simulink model "CTC_week5"  (Simulink 9.1)
settings: Solver=ode45  StartTime=0.0  StopTime=0.4  RelTol=1e-3  EnableMultiTasking=on
values from neighbouring files (symbols this model uses):
  g = 9.81    [project_week_5.m]
  h0 = thetaA_0(1)    [project_week_5.m]
  hm = thetaA_0(1)*0.5    [project_week_5.m]
  I_lower_xx = I_C(4)    [calculate_lagrange.m]    (also in calculate_lagrange_dependent.m; calculate_lagrange_fast.m; project_week_5.m = (1/12)*m_l*L(2)^2)
  I_lower_yy = I_C(5)    [calculate_lagrange.m]    (also in calculate_lagrange_dependent.m; calculate_lagrange_fast.m; project_week_5.m = (1/12)*m_l*L(2)^2)
  I_lower_zz = I_C(6)    [calculate_lagrange.m]    (also in calculate_lagrange_dependent.m; calculate_lagrange_fast.m; project_week_5.m = I_lower_xx/10)
  I_upper_xx = I_C(1)    [calculate_lagrange.m]    (also in calculate_lagrange_dependent.m; calculate_lagrange_fast.m; project_week_5.m = (1/12)*m_u*L(1)^2)
  I_upper_yy = I_C(2)    [calculate_lagrange.m]    (also in calculate_lagrange_dependent.m; calculate_lagrange_fast.m; project_week_5.m = (1/12)*m_u*L(1)^2)
  I_upper_zz = I_C(3)    [calculate_lagrange.m]    (also in calculate_lagrange_dependent.m; calculate_lagrange_fast.m; project_week_5.m = I_upper_xx/10)
  kc = M*wc^2*sqrt(alpha)    [project_week_5.m]
  L = [0.5,1,0.3,0.8]    [plot_inverse.m]    (also in project_week_5.m; project_week_5_boundaries.m = [0.8,1,0.4,0.5]; project_week_5_symbolic.m = [L_u L_l L_e L_b])
  m_l = 0.35    [project_week_5.m]
  m_p = 1    [project_week_5.m]
  m_u = 0.35    [project_week_5.m]
  q0d = q0(ind_d)    [project_week_5.m]
  q0i = q0(ind_i)    [project_week_5.m]
  R_L1_0 = R_L1_t(:,:,1)    [calculate_acceleration.m]    (also in calculate_position.m = R_L0(:,:,1); calculate_position_dep.m = R_L0(:,:,1); calculate_position_fast.m = R_L0(:,:,1); plot_inverse.m = R_A1*rot3D_Rodrigues([0;1;0],thetaL1_y_0))
  R_L2_0 = R_L2_t(:,:,1)    [calculate_acceleration.m]    (also in calculate_position.m = R_L0(:,:,2); calculate_position_dep.m = R_L0(:,:,2); calculate_position_fast.m = R_L0(:,:,2); plot_inverse.m = R_A2*rot3D_Rodrigues([0;1;0],thetaL2_y_0))
  R_L3_0 = R_L3_t(:,:,1)    [calculate_acceleration.m]    (also in calculate_position.m = R_L0(:,:,3); calculate_position_dep.m = R_L0(:,:,3); calculate_position_fast.m = R_L0(:,:,3); plot_inverse.m = R_A3*rot3D_Rodrigues([0;1;0],thetaL3_y_0))
  ti = beta*tz    [project_week_5.m]
  tm = cycleTime    (= 0.35)    [project_week_5.m]
  tp = alpha*tz    [project_week_5.m]
  tz = 1/(wc*sqrt(alpha))    [project_week_5.m]
undefined symbols (not defined in the file or in its folder): D, thetaU_0
(part 1 of 2)
settings Model: Creator=wouterh  LastModifiedBy=rober
settings DataIOCC: LimitDataPoints=on  SignalLoggingSaveFormat=ModelDataLogs
settings OptimizationCC: ExpressionDepthLimit=2147483647  InitFltsAndDblsToZero=on
settings DebuggingCC: SolverPrmCheckMsg=warning  FcnCallInpInsideContextMsg=warning  StateNameClashWarn=warning

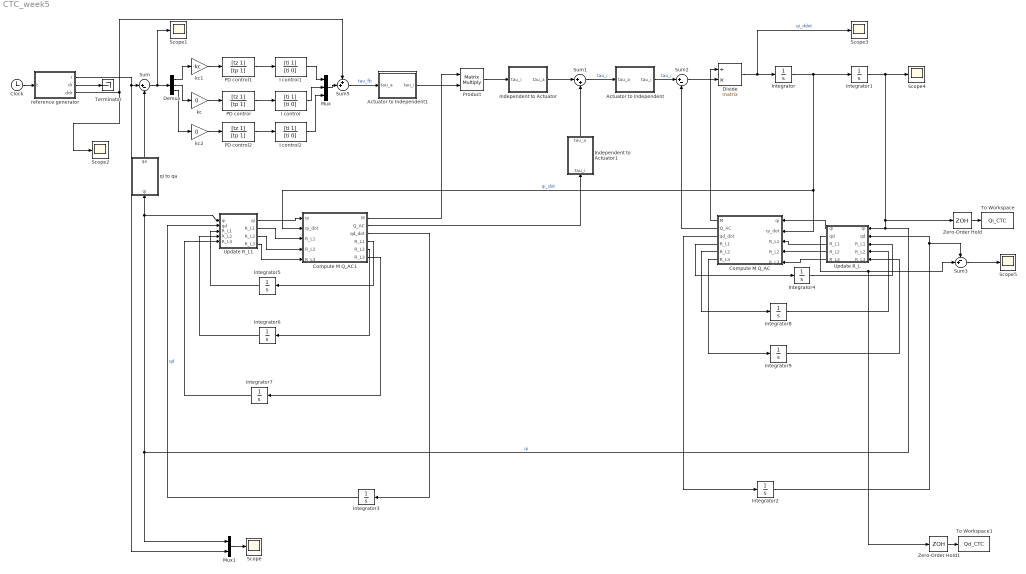
== system CTC_week5 ==
  Actuator to Independent : MATLAB Function  TreatAsAtomicUnit=on
  Actuator to Independent1 : MATLAB Function  TreatAsAtomicUnit=on
  Clock : Clock
  Compute M Q_AC : MATLAB Function  TreatAsAtomicUnit=on
  Compute M Q_AC1 : MATLAB Function  TreatAsAtomicUnit=on
  Demux : Demux  Outputs=3
  Divide : Product  Inputs=/*  Multiplication=Matrix(*)
  I control : TransferFcn  Numerator=[ti 1]  Denominator=[ti 0]
  I control1 : TransferFcn  Numerator=[ti 1]  Denominator=[ti 0]
  I control2 : TransferFcn  Numerator=[ti 1]  Denominator=[ti 0]
  Independent to Actuator : MATLAB Function  TreatAsAtomicUnit=on
  Independent to Actuator1 : MATLAB Function  TreatAsAtomicUnit=on
  Integrator : Integrator  InitialCondition=q0i
  Integrator1 : Integrator  InitialCondition=q0i
  Integrator2 : Integrator  InitialCondition=q0d
  Integrator3 : Integrator  InitialCondition=q0d
  Integrator4 : Integrator  InitialCondition=R_L1_0
  Integrator5 : Integrator  InitialCondition=R_L1_0
  Integrator6 : Integrator  InitialCondition=R_L2_0
  Integrator7 : Integrator  InitialCondition=R_L3_0
  Integrator8 : Integrator  InitialCondition=R_L2_0
  Integrator9 : Integrator  InitialCondition=R_L3_0
  Mux : Mux  Inputs=3
  Mux1 : Mux  Inputs=2
  PD control : TransferFcn  Numerator=[tz 1]  Denominator=[tp 1]
  PD control1 : TransferFcn  Numerator=[tz 1]  Denominator=[tp 1]
  PD control2 : TransferFcn  Numerator=[tz 1]  Denominator=[tp 1]
  Product : Product  Multiplication=Matrix(*)  RndMeth=Zero
  Scope{,1..5} (6 alike) : Scope
  Sum : Sum  Inputs=|+-
  Sum1 : Sum  Inputs=|++
  Sum2 : Sum  Inputs=|+-
  Sum3 : Sum  Inputs=-+|
  Sum5 : Sum  Inputs=++|
  Terminator : Terminator
  To Workspace : ToWorkspace  VariableName=Qi_CTC  SaveFormat=Timeseries  SampleTime=-1
  To Workspace1 : ToWorkspace  VariableName=Qd_CTC  SaveFormat=Timeseries  SampleTime=-1
  Update R_L : MATLAB Function  TreatAsAtomicUnit=on
  Update R_L1 : MATLAB Function  TreatAsAtomicUnit=on
  Zero-Order Hold : ZeroOrderHold  SampleTime=0.02
  Zero-Order Hold1 : ZeroOrderHold  SampleTime=0.02
  kc : Gain  Gain=0
  kc1 : Gain  Gain=-kc
  kc2 : Gain  Gain=0
  qi to qa : MATLAB Function  TreatAsAtomicUnit=on
  reference generator : MATLAB Function  TreatAsAtomicUnit=on
  wires:
  Clock/1 -> reference generator/1(t)
  reference generator/2(dr) -> Terminator/1
  reference generator/3(ddr) -> Sum5/1, Scope2/1
  Sum/1 -> Demux/1, Scope1/1
  PD control/1 -> I control/1
  Divide/1 -> Scope3/1, Integrator/1  "qi_ddot"
  Integrator/1 -> Integrator1/1, Compute M Q_AC1/2(qi_dot), Compute M Q_AC/2(qi_dot)  "qi_dot"
  Integrator1/1 -> Zero-Order Hold/1, Update R_L/1("qi "), qi to qa/1(qi), Update R_L1/1("qi "), Mux1/1, Scope4/1  "qi"
  Compute M Q_AC/1(M) -> Divide/1
  Compute M Q_AC1/2(Q_AC) -> Independent to Actuator1/1(tau_i)
  PD control1/1 -> I control1/1
  I control/1 -> Mux/2
  I control1/1 -> Mux/1
  Product/1 -> Independent to Actuator/1(tau_i)
  Mux/1 -> Sum5/2
  Sum5/1 -> Actuator to Independent1/1(tau_a)  "tau_fb"
  Mux1/1 -> Scope/1
  Compute M Q_AC/2(Q_AC) -> Sum2/2
  Compute M Q_AC/3(qd_dot) -> Integrator2/1
  Update R_L/1(qi) -> Compute M Q_AC/1(qi)
  Integrator2/1 -> Update R_L/2("qd "), Sum3/1
  kc1/1 -> PD control1/1
  Demux/1 -> kc1/1
  Demux/2 -> kc/1
  kc/1 -> PD control/1
  Sum3/1 -> Scope5/1
  reference generator/1(r) -> Mux1/2, Sum/1
  Zero-Order Hold/1 -> To Workspace/1
  Zero-Order Hold1/1 -> To Workspace1/1
  Update R_L/3(R_L1) -> Compute M Q_AC/3("R_L1 ")
  Compute M Q_AC/4(R_L1) -> Integrator4/1
  I control2/1 -> Mux/3
  kc2/1 -> PD control2/1
  PD control2/1 -> I control2/1
  Demux/3 -> kc2/1
  Update R_L1/1(qi) -> Compute M Q_AC1/1(qi)
  Update R_L1/2(R_L1) -> Compute M Q_AC1/3("R_L1 ")
  Compute M Q_AC1/4(R_L1) -> Integrator5/1
  Integrator3/1 -> Update R_L1/2(qd)  "qd"
  Sum2/1 -> Divide/2
  Actuator to Independent/1(tau_i) -> Sum2/1  "tau_i"
  qi to qa/1(qa) -> Sum/2
  Compute M Q_AC1/1(M) -> Product/1
  Sum1/1 -> Actuator to Independent/1(tau_a)  "tau_i"
  Independent to Actuator1/1(tau_a) -> Sum1/2
  Independent to Actuator/1(tau_a) -> Sum1/1
  Actuator to Independent1/1(tau_i) -> Product/2
  Compute M Q_AC1/5(R_L2) -> Integrator6/1
  Compute M Q_AC1/6(R_L3) -> Integrator7/1
  Compute M Q_AC/5(R_L2) -> Integrator8/1
  Compute M Q_AC/6(R_L3) -> Integrator9/1
  Integrator5/1 -> Update R_L1/3("R_L1 ")
  Integrator6/1 -> Update R_L1/4("R_L2 ")
  Integrator7/1 -> Update R_L1/5("R_L3 ")
  Integrator4/1 -> Update R_L/3("R_L1 ")
  Integrator8/1 -> Update R_L/4("R_L2 ")
  Integrator9/1 -> Update R_L/5("R_L3 ")
  Update R_L/2(qd) -> Zero-Order Hold1/1, Sum3/2
  Update R_L/4(R_L2) -> Compute M Q_AC/4("R_L2 ")
  Update R_L/5(R_L3) -> Compute M Q_AC/5("R_L3 ")
  Update R_L1/3(R_L2) -> Compute M Q_AC1/4("R_L2 ")
  Update R_L1/4(R_L3) -> Compute M Q_AC1/5("R_L3 ")
  Compute M Q_AC1/3(qd_dot) -> Integrator3/1

== matlab function Compute M Q_AC ==
  data: qi input double; qi_dot input double; R_L1 input double; R_L2 input double; R_L3 input double; M output double; Q_AC output double; m_u parameter double; m_p parameter double; m_l parameter double; L parameter double; D parameter double; g parameter double; qd_dot output double; R_L1 output double; I_upper_xx parameter double; I_upper_yy parameter double; I_upper_zz parameter double; I_lower_xx parameter double; I_lower_yy parameter double; I_lower_zz parameter double; thetaU_0 parameter double; R_L2 output double; R_L3 output double
function [M,Q_AC,qd_dot,R_L1,R_L2,R_L3] = fcn(qi,qi_dot,R_L1,R_L2,R_L3, m_u, m_p, m_l, L, D, g,I_upper_xx, I_upper_yy, I_upper_zz, I_lower_xx, I_lower_yy, I_lower_zz, thetaU_0)
% Compute dynamics for the system 
% Assume the model is perfect, so this is a copy past of M_Q_AC_model
% Requires running Project_week_4 first to get Mhat and Qhat


%Pre-initialise for Simulink
M=zeros(9,9);
Q_AC=zeros(9,1);
qd_dot=zeros(33,1);

%% Parameters
L_u=L(1);
L_l=L(2);
L_e=L(3);
thetaU1 = qi(1)/(+3^(1/2)/2) + thetaU_0(1); %qi()=thetaU1_x
thetaU2 = qi(4)/(-3^(1/2)/2) + thetaU_0(2); %qi()=thetaU2_x
thetaU3 = qi(8);                            %qi()=thetaU3_y
          
R_U1=rot3D_TaitByran(0, thetaU1, -2*pi/3);
R_U2=rot3D_TaitByran(0, thetaU2,  2*pi/3);
R_U3=rot3D_TaitByran(0, thetaU3,  0);
rL1_1_1 = R_L1(1,1); rL1_1_2 = R_L1(1,2); rL1_1_3 = R_L1(1,3);
rL1_2_1 = R_L1(2,1); rL1_2_2 = R_L1(2,2); rL1_2_3 = R_L1(2,3);
rL1_3_1 = R_L1(3,1); rL1_3_2 = R_L1(3,2); rL1_3_3 = R_L1(3,3);


rL2_1_1 = R_L2(1,1); rL2_1_2 = R_L2(1,2); rL2_1_3 = R_L2(1,3);
rL2_2_1 = R_L2(2,1); rL2_2_2 = R_L2(2,2); rL2_2_3 = R_L2(2,3);
rL2_3_1 = R_L2(3,1); rL2_3_2 = R_L2(3,2); rL2_3_3 = R_L2(3,3);

rL3_1_1 = R_L3(1,1); rL3_1_2 = R_L3(1,2); rL3_1_3 = R_L3(1,3);
rL3_2_1 = R_L3(2,1); rL3_2_2 = R_L3(2,2); rL3_2_3 = R_L3(2,3);
rL3_3_1 = R_L3(3,1); rL3_3_2 = R_L3(3,2); rL3_3_3 = R_L3(3,3);

%% Calculate moment inertias in the inertia frame
I_U1=R_U1*diag([I_upper_xx,I_upper_yy I_upper_zz])*R_U1.';
I_U2=R_U2*diag([I_upper_xx,I_upper_yy I_upper_zz])*R_U2.';
I_U3=R_U3*diag([I_upper_xx,I_upper_yy I_upper_zz])*R_U3.';

I_L1=R_L1*diag([I_lower_xx,I_lower_yy I_lower_zz])*R_L1.';
I_L2=R_L2*diag([I_lower_xx,I_lower_yy I_lower_zz])*R_L2.';
I_L3=R_L3*diag([I_lower_xx,I_lower_yy I_lower_zz])*R_L3.';

%% Partition into M*Qddot=[Mdd Mdi; Mid Mii]*[Qi_ddot Qd_ddot]
Mii = [I_U1 zeros(3,6);
      zeros(3,3) I_U2  zeros(3,3);
      zeros(3,6) I_U3];
Mdd = diag([0 0 0 ...
           m_u*[1 1 1]              ...
           m_l*[1 1 1] I_lower_xx I_lower_yy I_lower_zz ...
           m_u*[1 1 1]              ...
           m_l*[1 1 1] I_lower_xx I_lower_yy I_lower_zz ...
           m_u*[1 1 1]              ...
           m_l*[1 1 1] I_lower_xx I_lower_yy I_lower_zz ...
           m_p*[1 1 1] ]); 
% Correct Mdd
Mdd(10:12,10:12)=I_L1;
Mdd(19:21,19:21)=I_L2;
Mdd(28:30,28:30)=I_L3;
  
Mdi = zeros(33,9);
Mid = zeros(9,33);

%% function Jacobian_d = Jacobian_dNumeric(L_l,rL1_1_1,rL1_1_2,rL1_2_1,rL1_2_2,rL1_3_1,rL1_3_2,rL2_1_1,rL2_1_2,rL2_2_1,rL2_2_2,rL2_3_1,rL2_3_2,rL3_1_1,rL3_1_2,rL3_2_1,rL3_2_2,rL3_3_1,rL3_3_2)
%    This function was generated by the Symbolic Math Toolbox version 8.0.
t2 = L_l.*rL1_1_2.*rL1_2_1.*(1.0./2.0);
t3 = L_l.*rL1_1_2.*rL1_3_1.*(1.0./2.0);
t4 = L_l.*rL1_2_2.*rL1_3_1.*(1.0./2.0);
t5 = L_l.*rL1_1_1.*rL1_2_2.*(1.0./2.0);
t6 = L_l.*rL1_1_1.*rL1_3_2.*(1.0./2.0);
t7 = -t2+t5;
t8 = L_l.*rL1_2_1.*rL1_3_2.*(1.0./2.0);
t9 = -t3+t6;
t10 = -t4+t8;
t11 = L_l.*rL2_1_2.*rL2_2_1.*(1.0./2.0);
t12 = L_l.*rL2_1_2.*rL2_3_1.*(1.0./2.0);
t13 = L_l.*rL2_2_2.*rL2_3_1.*(1.0./2.0);
t14 = L_l.*rL2_1_1.*rL2_2_2.*(1.0./2.0);
t15 = L_l.*rL2_1_1.*rL2_3_2.*(1.0./2.0);
t16 = -t11+t14;
t17 = L_l.*rL2_2_1.*rL2_3_2.*(1.0./2.0);
t18 = -t12+t15;
t19 = -t13+t17;
t20 = L_l.*rL3_1_2.*rL3_2_1.*(1.0./2.0);
t21 = L_l.*rL3_1_2.*rL3_3_1.*(1.0./2.0);
t22 = L_l.*rL3_2_2.*rL3_3_1.*(1.0./2.0);
t23 = L_l.*rL3_1_1.*rL3_2_2.*(1.0./2.0);
t24 = L_l.*rL3_1_1.*rL3_3_2.*(1.0./2.0);
t25 = -t20+t23;
t26 = L_l.*rL3_2_1.*rL3_3_2.*(1.0./2.0);
t27 = -t21+t24;
t28 = -t22+t26;
t29 = sqrt(2.0);
t30 = sqrt(3.0);
Jacobian_d = reshape([1.0,0.0,0.0,0.0,0.0,0.0,0.0,0.0,0.0,1.0,0.0,0.0,0.0,0.0,0.0,0.0,0.0,0.0,1.0,0.0,0.0,0.0,0.0,0.0,0.0,0.0,0.0,1.0,0.0,0.0,0.0,0.0,0.0,0.0,1.0,0.0,0.0,0.0,0.0,0.0,0.0,0.0,0.0,1.0,0.0,0.0,0.0,0.0,0.0,0.0,0.0,0.0,1.0,0.0,0.0,0.0,0.0,0.0,0.0,0.0,0.0,1.0,0.0,0.0,0.0,0.0,0.0,0.0,1.0,0.0,0.0,0.0,0.0,0.0,0.0,0.0,0.0,1.0,0.0,0.0,0.0,0.0,0.0,0.0,0.0,0.0,1.0,0.0,0.0,0.0,0.0,0.0,0.0,0.0,0.0,1.0,0.0,0.0,0.0,-1.0,0.0,0.0,1.0,0.0,0.0,0.0,0.0,0.0,0.0,0.0,0.0,0.0,0.0,0.0,0.0,0.0,0.0,0.0,0.0,0.0,0.0,0.0,0.0,0.0,0.0,0.0,0.0,0.0,0.0,0.0,0.0,0.0,0.0,-1.0,0.0,0.0,1.0,0.0,0.0,0.0,0.0,0.0,0.0,0.0,0.0,0.0,0.0,0.0,0.0,0.0,0.0,0.0,0.0,0.0,0.0,0.0,0.0,0.0,0.0,0.0,0.0,0.0,0.0,0.0,0.0,0.0,0.0,-1.0,0.0,0.0,1.0,0.0,0.0,0.0,0.0,0.0,0.0,0.0,0.0,0.0,0.0,0.0,0.0,0.0,0.0,0.0,0.0,0.0,0.0,0.0,0.0,0.0,0.0,0.0,0.0,0.0,0.0,0.0,0.0,0.0,0.0,-1.0,0.0,0.0,1.0,0.0,0.0,0.0,0.0,0.0,0.0,0.0,0.0,0.0,0.0,0.0,0.0,0.0,0.0,0.0,0.0,0.0,0.0,0.0,0.0,0.0,0.0,0.0,0.0,0.0,0.0,0.0,0.0,0.0,0.0,-1.0,0.0,0.0,1.0,0.0,0.0,0.0,0.0,0.0,0.0,0.0,0.0,0.0,0.0,0.0,0.0,0.0,0.0,0.0,0.0,0.0,0.0,0.0,0.0,0.0,0.0,0.0,0.0,0.0,0.0,0.0,0.0,0.0,0.0,-1.0,0.0,0.0,1.0,0.0,0.0,0.0,0.0,0.0,0.0,0.0,0.0,0.0,0.0,0.0,0.0,0.0,0.0,0.0,0.0,0.0,0.0,0.0,0.0,0.0,0.0,0.0,0.0,0.0,0.0,0.0,0.0,t7,t9,0.0,t7,t9,0.0,0.0,0.0,0.0,0.0,0.0,0.0,0.0,0.0,0.0,0.0,0.0,0.0,0.0,0.0,0.0,0.0,0.0,0.0,0.0,0.0,rL1_2_2.*t29.*(-1.0./2.0)+rL1_3_2.*t29.*t30.*(1.0./4.0),0.0,0.0,0.0,0.0,0.0,t2-L_l.*rL1_1_1.*rL1_2_2.*(1.0./2.0),0.0,t10,t2-t5,0.0,t10,0.0,0.0,0.0,0.0,0.0,0.0,0.0,0.0,0.0,0.0,0.0,0.0,0.0,0.0,0.0,0.0,0.0,0.0,0.0,0.0,0.0,rL1_1_2.*t29.*(1.0./2.0)-rL1_3_2.*t29.*(1.0./4.0),0.0,0.0,0.0,0.0,0.0,t3-L_l.*rL1_1_1.*rL1_3_2.*(1.0./2.0),t4-L_l.*rL1_2_1.*rL1_3_2.*(1.0./2.0),0.0,t3-t6,t4-t8,0.0,0.0,0.0,0.0,0.0,0.0,0.0,0.0,0.0,0.0,0.0,0.0,0.0,0.0,0.0,0.0,0.0,0.0,0.0,0.0,0.0,0.0,rL1_2_2.*t29.*(1.0./4.0)-rL1_1_2.*t29.*t30.*(1.0./4.0),0.0,0.0,0.0,0.0,0.0,0.0,0.0,0.0,0.0,0.0,0.0,-1.0,0.0,0.0,1.0,0.0,0.0,0.0,0.0,0.0,0.0,0.0,0.0,0.0,0.0,0.0,0.0,0.0,0.0,0.0,0.0,0.0,0.0,0.0,0.0,0.0,0.0,0.0,0.0,0.0,0.0,0.0,0.0,0.0,0.0,-1.0,0.0,0.0,1.0,0.0,0.0,0.0,0.0,0.0,0.0,0.0,0.0,0.0,0.0,0.0,0.0,0.0,0.0,0.0,0.0,0.0,0.0,0.0,0.0,0.0,0.0,0.0,0.0,0.0,0.0,0.0,0.0,0.0,0.0,-1.0,0.0,0.0,1.0,0.0,0.0,0.0,0.0,0.0,0.0,0.0,0.0,0.0,0.0,0.0,0.0,0.0,0.0,0.0,0.0,0.0,0.0,0.0,0.0,0.0,0.0,0.0,0.0,0.0,0.0,0.0,0.0,0.0,0.0,-1.0,0.0,0.0,1.0,0.0,0.0,0.0,0.0,0.0,0.0,0.0,0.0,0.0,0.0,0.0,0.0,0.0,0.0,0.0,0.0,0.0,0.0,0.0,0.0,0.0,0.0,0.0,0.0,0.0,0.0,0.0,0.0,0.0,0.0,-1.0,0.0,0.0,1.0,0.0,0.0,0.0,0.0,0.0,0.0,0.0,0.0,0.0,0.0,0.0,0.0,0.0,0.0,0.0,0.0,0.0,0.0,0.0,0.0,0.0,0.0,0.0,0.0,0.0,0.0,0.0,0.0,0.0,0.0,-1.0,0.0,0.0,1.0,0.0,0.0,0.0,0.0,0.0,0.0,0.0,0.0,0.0,0.0,0.0,0.0,0.0,0.0,0.0,0.0,0.0,0.0,0.0,0.0,0.0,0.0,0.0,0.0,0.0,0.0,0.0,0.0,t16,t18,0.0,t16,t18,0.0,0.0,0.0,0.0,0.0,0.0,0.0,0.0,0.0,0.0,0.0,0.0,0.0,rL2_2_2.*t29.*(-1.0./2.0)-rL2_3_2.*t29.*t30.*(1.0./4.0),0.0,0.0,0.0,0.0,0.0,0.0,0.0,0.0,0.0,0.0,0.0,0.0,0.0,t11-L_l.*rL2_1_1.*rL2_2_2.*(1.0./2.0),0.0,t19,t11-t14,0.0,t19,0.0,0.0,0.0,0.0,0.0,0.0,0.0,0.0,0.0,0.0,0.0,0.0,0.0,rL2_1_2.*t29.*(1.0./2.0)-rL2_3_2.*t29.*(1.0./4.0),0.0,0.0,0.0,0.0,0.0,0.0,0.0,0.0,0.0,0.0,0.0,0.0,0.0,t12-L_l.*rL2_1_1.*rL2_3_2.*(1.0./2.0),t13-L_l.*rL2_2_1.*rL2_3_2.*(1.0./2.0),0.0,t12-t15,t13-t17,0.0,0.0,0.0,0.0,0.0,0.0,0.0,0.0,0.0,0.0,0.0,0.0,0.0,0.0,rL2_2_2.*t29.*(1.0./4.0)+rL2_1_2.*t29.*t30.*(1.0./4.0),0.0,0.0,0.0,0.0,0.0,0.0,0.0,0.0,0.0,0.0,0.0,0.0,0.0,0.0,0.0,0.0,0.0,0.0,0.0,-1.0,0.0,0.0,1.0,0.0,0.0,0.0,0.0,0.0,0.0,0.0,0.0,0.0,0.0,0.0,0.0,0.0,0.0,0.0,0.0,0.0,0.0,0.0,0.0,0.0,0.0,0.0,0.0,0.0,0.0,0.0,0.0,0.0,0.0,-1.0,0.0,0.0,1.0,0.0,0.0,0.0,0.0,0.0,0.0,0.0,0.0,0.0,0.0,0.0,0.0,0.0,0.0,0.0,0.0,0.0,0.0,0.0,0.0,0.0,0.0,0.0,0.0,0.0,0.0,0.0,0.0,0.0,0.0,-1.0,0.0,0.0,1.0,0.0,0.0,0.0,0.0,0.0,0.0,0.0,0.0,0.0,0.0,0.0,0.0,0.0,0.0,0.0,0.0,0.0,0.0,0.0,0.0,0.0,0.0,0.0,0.0,0.0,0.0,0.0,0.0,0.0,0.0,-1.0,0.0,0.0,1.0,0.0,0.0,0.0,0.0,0.0,0.0,0.0,0.0,0.0,0.0,0.0,0.0,0.0,0.0,0.0,0.0,0.0,0.0,0.0,0.0,0.0,0.0,0.0,0.0,0.0,0.0,0.0,0.0,0.0,0.0,-1.0,0.0,0.0,1.0,0.0,0.0,0.0,0.0,0.0,0.0,0.0,0.0,0.0,0.0,0.0,0.0,0.0,0.0,0.0,0.0,0.0,0.0,0.0,0.0,0.0,0.0,0.0,0.0,0.0,0.0,0.0,0.0,0.0,0.0,-1.0,0.0,0.0,1.0,0.0,0.0,0.0,0.0,0.0,0.0,0.0,0.0,0.0,0.0,0.0,0.0,0.0,0.0,0.0,0.0,0.0,0.0,0.0,0.0,0.0,0.0,0.0,0.0,0.0,0.0,0.0,0.0,t25,t27,0.0,t25,t27,0.0,0.0,0.0,0.0,0.0,rL3_2_2.*t29.*(-1.0./2.0),0.0,0.0,0.0,0.0,0.0,0.0,0.0,0.0,0.0,0.0,0.0,0.0,0.0,0.0,0.0,0.0,0.0,0.0,0.0,0.0,0.0,t20-L_l.*rL3_1_1.*rL3_2_2.*(1.0./2.0),0.0,t28,t20-t23,0.0,t28,0.0,0.0,0.0,0.0,0.0,rL3_1_2.*t29.*(1.0./2.0)+rL3_3_2.*t29.*(1.0./2.0),0.0,0.0,0.0,0.0,0.0,0.0,0.0,0.0,0.0,0.0,0.0,0.0,0.0,0.0,0.0,0.0,0.0,0.0,0.0,0.0,0.0,t21-L_l.*rL3_1_1.*rL3_3_2.*(1.0./2.0),t22-L_l.*rL3_2_1.*rL3_3_2.*(1.0./2.0),0.0,t21-t24,t22-t26,0.0,0.0,0.0,0.0,0.0,0.0,rL3_2_2.*t29.*(-1.0./2.0),0.0,0.0,0.0,0.0,0.0,0.0,-1.0,0.0,0.0,0.0,0.0,0.0,0.0,0.0,0.0,-1.0,0.0,0.0,0.0,0.0,0.0,0.0,0.0,0.0,-1.0,0.0,0.0,0.0,0.0,0.0,0.0,0.0,0.0,0.0,0.0,0.0,0.0,0.0,0.0,0.0,-1.0,0.0,0.0,0.0,0.0,0.0,0.0,0.0,0.0,-1.0,0.0,0.0,0.0,0.0,0.0,0.0,0.0,0.0,-1.0,0.0,0.0,0.0,0.0,0.0,0.0,0.0,0.0,0.0,0.0,0.0,0.0,0.0,0.0,0.0,-1.0,0.0,0.0,0.0,0.0,0.0,0.0,0.0,0.0,-1.0,0.0,0.0,0.0,0.0,0.0,0.0,0.0,0.0,-1.0,0.0,0.0,0.0,0.0,0.0,0.0],[33,33]);

%% function Jacobian_i = Jacobian_iNumeric(L_u,thetaU1,thetaU2,thetaU3)
t2 = cos(thetaU1);
t3 = sin(thetaU1);
t4 = sqrt(3.0);
t5 = L_u.*t3.*(1.0./4.0);
t6 = L_u.*t2.*(1.0./2.0);
t7 = L_u.*t3.*t4.*(1.0./4.0);
t8 = cos(thetaU2);
t9 = sin(thetaU2);
t10 = L_u.*t4.*t9.*(1.0./4.0);
t11 = L_u.*t9.*(1.0./4.0);
t12 = L_u.*t8.*(1.0./2.0);
t13 = cos(thetaU3);
t14 = sin(thetaU3);
t15 = L_u.*t13.*(1.0./2.0);
t16 = L_u.*t14.*(1.0./2.0);
Jacobian_i = reshape([0.0,t6,t7,0.0,t6,t7,0.0,0.0,0.0,0.0,0.0,0.0,0.0,0.0,0.0,0.0,0.0,0.0,0.0,0.0,0.0,0.0,0.0,0.0,0.0,0.0,0.0,0.0,0.0,0.0,0.0,0.0,0.0,L_u.*t2.*(-1.0./2.0),0.0,-t5,-t6,0.0,-t5,0.0,0.0,0.0,0.0,0.0,0.0,0.0,0.0,0.0,0.0,0.0,0.0,0.0,0.0,0.0,0.0,0.0,0.0,0.0,0.0,0.0,0.0,0.0,0.0,0.0,0.0,0.0,L_u.*t3.*t4.*(-1.0./4.0),t5,0.0,-t7,t5,0.0,0.0,0.0,0.0,0.0,0.0,0.0,0.0,0.0,0.0,0.0,0.0,0.0,0.0,0.0,0.0,0.0,0.0,0.0,0.0,0.0,0.0,0.0,0.0,0.0,0.0,0.0,0.0,0.0,0.0,0.0,0.0,0.0,0.0,0.0,0.0,0.0,0.0,t12,-t10,0.0,t12,-t10,0.0,0.0,0.0,0.0,0.0,0.0,0.0,0.0,0.0,0.0,0.0,0.0,0.0,0.0,0.0,0.0,0.0,0.0,0.0,0.0,0.0,0.0,0.0,0.0,0.0,0.0,0.0,L_u.*t8.*(-1.0./2.0),0.0,-t11,-t12,0.0,-t11,0.0,0.0,0.0,0.0,0.0,0.0,0.0,0.0,0.0,0.0,0.0,0.0,0.0,0.0,0.0,0.0,0.0,0.0,0.0,0.0,0.0,0.0,0.0,0.0,0.0,0.0,0.0,t10,t11,0.0,t10,t11,0.0,0.0,0.0,0.0,0.0,0.0,0.0,0.0,0.0,0.0,0.0,0.0,0.0,0.0,0.0,0.0,0.0,0.0,0.0,0.0,0.0,0.0,0.0,0.0,0.0,0.0,0.0,0.0,0.0,0.0,0.0,0.0,0.0,0.0,0.0,0.0,0.0,0.0,t15,0.0,0.0,t15,0.0,0.0,0.0,0.0,0.0,0.0,0.0,0.0,0.0,0.0,0.0,0.0,0.0,0.0,0.0,0.0,0.0,0.0,0.0,0.0,0.0,0.0,0.0,0.0,0.0,0.0,0.0,0.0,L_u.*t13.*(-1.0./2.0),0.0,t16,-t15,0.0,t16,0.0,0.0,0.0,0.0,0.0,0.0,0.0,0.0,0.0,0.0,0.0,0.0,0.0,0.0,0.0,0.0,0.0,0.0,0.0,0.0,0.0,0.0,0.0,0.0,0.0,0.0,0.0,0.0,L_u.*t14.*(-1.0./2.0),0.0,0.0,-t16,0.0,0.0,0.0,0.0,0.0,0.0,0.0,0.0,0.0,0.0],[33,9]);

%% Compute dependent velocities
P = Jacobian_d\Jacobian_i;
Phi_t=zeros(33,1);
qd_dot = -P*qi_dot-Jacobian_d\Phi_t;

qdot=[qd_dot(1:6); qi_dot(1:3);qd_dot(7:16);qi_dot(4:6);qd_dot(17:26);qi_dot(7:9);qd_dot(27:33)];
qdot1=qdot(1);
qdot2=qdot(2);
qdot3=qdot(3);
qdot4=qdot(4);
qdot5=qdot(5);
qdot6=qdot(6);
qdot7=qdot(7);
qdot8=qdot(8);
qdot9=qdot(9);
qdot10=qdot(10);
qdot11=qdot(11);
qdot12=qdot(12);
qdot13=qdot(13);
qdot14=qdot(14);
qdot15=qdot(15);
qdot16=qdot(16);
qdot17=qdot(17);
qdot18=qdot(18);
qdot19=qdot(19);
qdot20=qdot(20);
qdot21=qdot(21);
qdot22=qdot(22);
qdot23=qdot(23);
qdot24=qdot(24);
qdot25=qdot(25);
qdot26=qdot(26);
qdot27=qdot(27);
qdot28=qdot(28);
qdot29=qdot(29);
qdot30=qdot(30);
qdot31=qdot(31);
qdot32=qdot(32);
qdot33=qdot(33);
qdot34=qdot(34);
qdot35=qdot(35);
qdot36=qdot(36);
qdot37=qdot(37);
qdot38=qdot(38);
qdot39=qdot(39);
qdot40=qdot(40);
qdot41=qdot(41);
qdot42=qdot(42);
%% function Gamma_without_driving = Gamma_without_drivingNumeric(L_l,L_u,qdot7,qdot8,qdot9,qdot13,qdot14,qdot15,qdot19,qdot20,qdot21,qdot25,qdot26,qdot27,qdot31,qdot32,qdot33,qdot37,qdot38,qdot39,rL1_1_1,rL1_1_2,rL1_1_3,rL1_2_1,rL1_2_2,rL1_2_3,rL1_3_1,rL1_3_2,rL1_3_3,rL2_1_1,rL2_1_2,rL2_1_3,rL2_2_1,rL2_2_2,rL2_2_3,rL2_3_1,rL2_3_2,rL2_3_3,rL3_1_1,rL3_1_2,rL3_1_3,rL3_2_1,rL3_2_2,rL3_2_3,rL3_3_1,rL3_3_2,rL3_3_3,thetaU1,thetaU2,thetaU3)
%    This function was generated by the Symbolic Math Toolbox version 8.0.
t2 = sqrt(3.0);
t3 = cos(thetaU1);
t4 = sin(thetaU1);
t5 = qdot8.*t4;
t22 = qdot9.*t2.*t3.*(1.0./2.0);
t6 = t5-t22;
t7 = L_u.*qdot9.*t2.*t3.*(1.0./8.0);
t8 = qdot7.*t4;
t33 = qdot9.*t3.*(1.0./2.0);
t9 = t8-t33;
t10 = qdot9.^2;
t11 = qdot8.*t3.*(1.0./2.0);
t38 = qdot7.*t2.*t3.*(1.0./2.0);
t12 = t11-t38;
t13 = qdot7.*(1.0./2.0);
t14 = qdot8.*t2.*(1.0./2.0);
t15 = t13+t14;
t16 = qdot15.*rL1_2_1;
t20 = qdot14.*rL1_3_1;
t17 = t16-t20;
t18 = qdot15.*rL1_2_2;
t21 = qdot14.*rL1_3_2;
t19 = t18-t21;
t23 = L_u.*qdot9.*t3.*(1.0./8.0);
t24 = t23-L_u.*t2.*t6.*(1.0./4.0);
t25 = L_u.*t6.*(1.0./4.0);
t26 = t7+t25;
t27 = qdot15.*rL1_1_1;
t31 = qdot13.*rL1_3_1;
t28 = t27-t31;
t29 = qdot15.*rL1_1_2;
t32 = qdot13.*rL1_3_2;
t30 = t29-t32;
t34 = L_u.*t2.*t9.*(1.0./4.0);
t35 = t7+t34;
t36 = L_u.*t9.*(1.0./4.0);
t37 = qdot8.*(t36-L_u.*qdot9.*t3.*(3.0./8.0));
t39 = L_u.*t2.*t12.*(1.0./4.0);
t40 = t39-L_u.*t3.*t15.*(1.0./4.0);
t41 = L_u.*t12.*(1.0./4.0);
t42 = L_u.*t2.*t3.*t15.*(1.0./4.0);
t43 = t41+t42;
t44 = qdot8.*t43;
t45 = qdot14.*rL1_1_1;
t49 = qdot13.*rL1_2_1;
t46 = t45-t49;
t47 = qdot14.*rL1_1_2;
t50 = qdot13.*rL1_2_2;
t48 = t47-t50;
t51 = L_u.*qdot9.*t4.*t15.*(1.0./2.0);
t52 = L_l.*rL1_1_2.*t17.*(1.0./2.0);
t53 = t52-L_l.*rL1_1_1.*t19.*(1.0./2.0);
t54 = qdot13.*t53;
t55 = L_l.*rL1_2_2.*t17.*(1.0./2.0);
t56 = t55-L_l.*rL1_2_1.*t19.*(1.0./2.0);
t57 = qdot14.*t56;
t58 = L_l.*rL1_3_2.*t17.*(1.0./2.0);
t59 = t58-L_l.*rL1_3_1.*t19.*(1.0./2.0);
t60 = qdot15.*t59;
t61 = L_l.*rL1_1_2.*t28.*(1.0./2.0);
t62 = t61-L_l.*rL1_1_1.*t30.*(1.0./2.0);
t63 = L_l.*rL1_2_2.*t28.*(1.0./2.0);
t64 = t63-L_l.*rL1_2_1.*t30.*(1.0./2.0);
t65 = L_l.*rL1_3_2.*t28.*(1.0./2.0);
t66 = t65-L_l.*rL1_3_1.*t30.*(1.0./2.0);
t67 = L_l.*rL1_1_2.*t46.*(1.0./2.0);
t68 = t67-L_l.*rL1_1_1.*t48.*(1.0./2.0);
t69 = qdot13.*t68;
t70 = L_l.*rL1_2_2.*t46.*(1.0./2.0);
t71 = t70-L_l.*rL1_2_1.*t48.*(1.0./2.0);
t72 = qdot14.*t71;
t73 = L_l.*rL1_3_2.*t46.*(1.0./2.0);
t74 = t73-L_l.*rL1_3_1.*t48.*(1.0./2.0);
t75 = qdot15.*t74;
t76 = cos(thetaU2);
t77 = sin(thetaU2);
t78 = qdot20.*t77;
t79 = qdot21.*t2.*t76.*(1.0./2.0);
t80 = t78+t79;
t81 = qdot19.*t77;
t107 = qdot21.*t76.*(1.0./2.0);
t82 = t81-t107;
t83 = qdot21.^2;
t84 = qdot20.*t76.*(1.0./2.0);
t85 = qdot19.*t2.*t76.*(1.0./2.0);
t86 = t84+t85;
t87 = qdot19.*(1.0./2.0);
t89 = qdot20.*t2.*(1.0./2.0);
t88 = t87-t89;
t90 = qdot27.*rL2_2_1;
t94 = qdot26.*rL2_3_1;
t91 = t90-t94;
t92 = qdot27.*rL2_2_2;
t95 = qdot26.*rL2_3_2;
t93 = t92-t95;
t96 = L_u.*t2.*t80.*(1.0./4.0);
t97 = L_u.*qdot21.*t76.*(1.0./8.0);
t98 = t96+t97;
t99 = L_u.*t80.*(1.0./4.0);
t100 = L_u.*qdot21.*t2.*t76.*(1.0./8.0);
t101 = qdot27.*rL2_1_1;
t105 = qdot25.*rL2_3_1;
t102 = t101-t105;
t103 = qdot27.*rL2_1_2;
t106 = qdot25.*rL2_3_2;
t104 = t103-t106;
t108 = L_u.*t2.*t82.*(1.0./4.0);
t109 = qdot19.*(t100+t108);
t110 = L_u.*t82.*(1.0./4.0);
t111 = qdot20.*(t110-L_u.*qdot21.*t76.*(3.0./8.0));
t112 = L_u.*t2.*t77.*t83.*(1.0./4.0);
t113 = L_u.*t2.*t86.*(1.0./4.0);
t114 = L_u.*t76.*t88.*(1.0./4.0);
t115 = t113+t114;
t116 = qdot19.*t115;
t117 = L_u.*t86.*(1.0./4.0);
t118 = t117-L_u.*t2.*t76.*t88.*(1.0./4.0);
t119 = qdot20.*t118;
t120 = qdot26.*rL2_1_1;
t124 = qdot25.*rL2_2_1;
t121 = t120-t124;
t122 = qdot26.*rL2_1_2;
t125 = qdot25.*rL2_2_2;
t123 = t122-t125;
t126 = L_u.*qdot21.*t77.*t88.*(1.0./2.0);
t127 = L_l.*rL2_1_2.*t91.*(1.0./2.0);
t128 = t127-L_l.*rL2_1_1.*t93.*(1.0./2.0);
t129 = qdot25.*t128;
t130 = L_l.*rL2_2_2.*t91.*(1.0./2.0);
t131 = t130-L_l.*rL2_2_1.*t93.*(1.0./2.0);
t132 = qdot26.*t131;
t133 = L_l.*rL2_3_2.*t91.*(1.0./2.0);
t134 = t133-L_l.*rL2_3_1.*t93.*(1.0./2.0);
t135 = qdot27.*t134;
t136 = L_l.*rL2_1_2.*t102.*(1.0./2.0);
t137 = t136-L_l.*rL2_1_1.*t104.*(1.0./2.0);
t138 = L_l.*rL2_2_2.*t102.*(1.0./2.0);
t139 = t138-L_l.*rL2_2_1.*t104.*(1.0./2.0);
t140 = L_l.*rL2_3_2.*t102.*(1.0./2.0);
t141 = t140-L_l.*rL2_3_1.*t104.*(1.0./2.0);
t142 = L_l.*rL2_1_2.*t121.*(1.0./2.0);
t143 = t142-L_l.*rL2_1_1.*t123.*(1.0./2.0);
t144 = qdot25.*t143;
t145 = L_l.*rL2_2_2.*t121.*(1.0./2.0);
t146 = t145-L_l.*rL2_2_1.*t123.*(1.0./2.0);
t147 = qdot26.*t146;
t148 = L_l.*rL2_3_2.*t121.*(1.0./2.0);
t149 = t148-L_l.*rL2_3_1.*t123.*(1.0./2.0);
t150 = qdot27.*t149;
t151 = sin(thetaU3);
t152 = cos(thetaU3);
t153 = qdot32.^2;
t154 = qdot39.*rL3_2_1;
t158 = qdot38.*rL3_3_1;
t155 = t154-t158;
t156 = qdot39.*rL3_2_2;
t159 = qdot38.*rL3_3_2;
t157 = t156-t159;
t160 = L_u.*t151.*t153.*(1.0./2.0);
t161 = qdot33.^2;
t162 = L_u.*t151.*t161.*(1.0./2.0);
t163 = qdot39.*rL3_1_1;
t167 = qdot37.*rL3_3_1;
t164 = t163-t167;
t165 = qdot39.*rL3_1_2;
t168 = qdot37.*rL3_3_2;
t166 = t165-t168;
t169 = qdot33.*t152;
t170 = qdot31.*t151;
t171 = t169+t170;
t172 = qdot38.*rL3_1_1;
t176 = qdot37.*rL3_2_1;
t173 = t172-t176;
t174 = qdot38.*rL3_1_2;
t177 = qdot37.*rL3_2_2;
t175 = t174-t177;
t178 = qdot31.^2;
t179 = L_u.*t152.*t178.*(1.0./2.0);
t180 = L_u.*t152.*t153.*(1.0./2.0);
t181 = L_l.*rL3_1_2.*t155.*(1.0./2.0);
t182 = t181-L_l.*rL3_1_1.*t157.*(1.0./2.0);
t183 = qdot37.*t182;
t184 = L_l.*rL3_2_2.*t155.*(1.0./2.0);
t185 = t184-L_l.*rL3_2_1.*t157.*(1.0./2.0);
t186 = qdot38.*t185;
t187 = L_l.*rL3_3_2.*t155.*(1.0./2.0);
t188 = t187-L_l.*rL3_3_1.*t157.*(1.0./2.0);
t189 = qdot39.*t188;
t190 = L_l.*rL3_1_2.*t164.*(1.0./2.0);
t191 = t190-L_l.*rL3_1_1.*t166.*(1.0./2.0);
t192 = L_l.*rL3_2_2.*t164.*(1.0./2.0);
t193 = t192-L_l.*rL3_2_1.*t166.*(1.0./2.0);
t194 = L_l.*rL3_3_2.*t164.*(1.0./2.0);
t195 = t194-L_l.*rL3_3_1.*t166.*(1.0./2.0);
t196 = L_l.*rL3_1_2.*t173.*(1.0./2.0);
t197 = t196-L_l.*rL3_1_1.*t175.*(1.0./2.0);
t198 = qdot37.*t197;
t199 = L_l.*rL3_2_2.*t173.*(1.0./2.0);
t200 = t199-L_l.*rL3_2_1.*t175.*(1.0./2.0);
t201 = qdot38.*t200;
t202 = L_l.*rL3_3_2.*t173.*(1.0./2.0);
t203 = t202-L_l.*rL3_3_1.*t175.*(1.0./2.0);
t204 = qdot39.*t203;
t205 = sqrt(2.0);
t206 = t16-qdot13.*rL1_2_3;
t207 = qdot13.*rL1_3_3;
t208 = t207-qdot15.*rL1_3_1;
t209 = t101-qdot25.*rL2_1_3;
t210 = t90-qdot25.*rL2_2_3;
t211 = qdot25.*rL2_3_3;
t212 = t211-qdot27.*rL2_3_1;
t213 = t154-qdot37.*rL3_2_3;
Gamma_without_driving = [-qdot7.*t24-qdot8.*t26-L_u.*t4.*t10.*(1.0./4.0);t37-qdot7.*t35-L_u.*t2.*t4.*t10.*(1.0./4.0);t44+t51-qdot7.*t40;t54+t57+t60-qdot7.*t24-qdot8.*t26-L_u.*t4.*t10.*(1.0./4.0);t37-qdot7.*t35-qdot13.*t62-qdot14.*t64-qdot15.*t66-L_u.*t2.*t4.*t10.*(1.0./4.0);t44+t51+t69+t72+t75-qdot7.*t40;t54+t57+t60;-qdot13.*t62-qdot14.*t64-qdot15.*t66;t69+t72+t75;-qdot19.*t98-qdot20.*(t99-L_u.*qdot21.*t2.*t76.*(1.0./8.0))-L_u.*t77.*t83.*(1.0./4.0);t109+t111+t112;t116+t119+t126;t129+t132+t135-qdot19.*t98-qdot20.*(t99-t100)-L_u.*t77.*t83.*(1.0./4.0);t109+t111+t112-qdot25.*t137-qdot26.*t139-qdot27.*t141;t116+t119+t126+t144+t147+t150;t129+t132+t135;-qdot25.*t137-qdot26.*t139-qdot27.*t141;t144+t147+t150;t160+t162-L_u.*qdot31.*qdot33.*t152.*(1.0./2.0);L_u.*qdot32.*t171.*(-1.0./2.0);t179+t180-L_u.*qdot31.*qdot33.*t151.*(1.0./2.0);t160+t162+t183+t186+t189-L_u.*qdot31.*qdot33.*t152.*(1.0./2.0);-qdot37.*t191-qdot38.*t193-qdot39.*t195-L_u.*qdot32.*t171.*(1.0./2.0);t179+t180+t198+t201+t204-L_u.*qdot31.*qdot33.*t151.*(1.0./2.0);t183+t186+t189;-qdot37.*t191-qdot38.*t193-qdot39.*t195;t198+t201+t204;0.0;0.0;0.0;-qdot13.*(t205.*t206.*(1.0./2.0)+t2.*t205.*t208.*(1.0./4.0))+qdot14.*(t205.*t208.*(1.0./4.0)+t205.*(t27-qdot13.*rL1_1_3).*(1.0./2.0))+qdot15.*(t205.*t206.*(1.0./4.0)-t2.*t205.*(t27-qdot13.*rL1_1_3).*(1.0./4.0));-qdot25.*(t205.*t210.*(1.0./2.0)-t2.*t205.*t212.*(1.0./4.0))+qdot27.*(t205.*t210.*(1.0./4.0)+t2.*t205.*t209.*(1.0./4.0))+qdot26.*(t205.*t209.*(1.0./2.0)+t205.*t212.*(1.0./4.0));-qdot38.*(t205.*(qdot37.*rL3_3_3-qdot39.*rL3_3_1).*(1.0./2.0)-t205.*(t163-qdot37.*rL3_1_3).*(1.0./2.0))-qdot37.*t205.*t213.*(1.0./2.0)-qdot39.*t205.*t213.*(1.0./2.0)];

%% Compute QAi and QAd
QAd=zeros(33,1);
% Gravity
QAd(6)=-m_u*g;
QAd(9)=-m_l*g;
QAd(15)=-m_u*g;
QAd(18)=-m_l*g;
QAd(24)=-m_u*g;
QAd(27)=-m_l*g;
QAd(33)=-m_p*g;

% Calculate gyroscopic forces in the inertia frame
C_U1=R_U1*tilde(qdot(7:9))*diag([I_upper_xx,I_upper_yy I_upper_zz])*R_U1.'*qdot(7:9);
C_U2=R_U2*tilde(qdot(19:21))*diag([I_upper_xx,I_upper_yy I_upper_zz])*R_U2.'*qdot(19:21);
C_U3=R_U3*tilde(qdot(31:33))*diag([I_upper_xx,I_upper_yy I_upper_zz])*R_U3.'*qdot(31:33);

C_L1=R_L1*tilde(qdot(13:15))*diag([I_lower_xx,I_lower_yy I_lower_zz])*R_L1.'*qdot(13:15);
C_L2=R_L2*tilde(qdot(25:27))*diag([I_lower_xx,I_lower_yy I_lower_zz])*R_L2.'*qdot(25:27);
C_L3=R_L3*tilde(qdot(37:39))*diag([I_lower_xx,I_lower_yy I_lower_zz])*R_L3.'*qdot(37:39);

% dependent C, lower angles
QAd(10:12)=C_L1;  
QAd(19:21)=C_L2;
QAd(28:30)=C_L3;

% independent C
QAi=zeros(9,1);
QAi(1:3)=C_U1;
QAi(4:6)=C_U2;
QAi(7:9)=C_U3;
%% Compute Ouputs
P2 = Jacobian_d\Gamma_without_driving;

M = Mii - Mid*P - P.'*(Mdi - Mdd*P); 
Q_AC = QAi-Mid*P2 -P.'*QAd +  P.'*Mdd*P2;

end

== matlab function Update R_L ==
  data: qi input double; qi output double; qd input double; qd output double; L parameter double; D parameter double; R_L1 input double; R_L2 input double; R_L3 input double; R_L1 output double; R_L1_0 parameter double; R_L2_0 parameter double; R_L3_0 parameter double; thetaU_0 parameter double; R_L2 output double; R_L3 output double
function [qi,qd,R_L1,R_L2,R_L3] = fcn(qi,qd,L, D,R_L1,R_L2,R_L3,R_L1_0, R_L2_0, R_L3_0, thetaU_0)
% Compute dynamics for the system 
% Assume the model is perfect, so this is a copy past of M_Q_AC_model
% Requires running Project_week_4 first to get Mhat and Qhat


%Pre-initialise for Simulink
L_u=L(1);
L_l=L(2);
L_e=L(3);
tolerance=0.0001;


thetaU1 = qi(1)/(+3^(1/2)/2) + thetaU_0(1); %qi()=thetaU1_x
thetaU2 = qi(4)/(-3^(1/2)/2) + thetaU_0(2); %qi()=thetaU2_x
thetaU3 = qi(8);                            %qi()=thetaU3_y

R_U1=rot3D_TaitByran(0, thetaU1, -2*pi/3);
R_U2=rot3D_TaitByran(0, thetaU2, +2*pi/3);
R_U3=rot3D_TaitByran(0, thetaU3,  0);
R_A1=rot3D_TaitByran(0, 0, -2*pi/3); % constant
R_A2=rot3D_TaitByran(0, 0, +2*pi/3); % constant
R_A3=rot3D_TaitByran(0, 0, 0); % constant
% 
% if time == 0
%    %q=q0;
%    R_L(:,:,1) = R_L1_0; 
%    R_L(:,:,2) = R_L2_0; 
%    R_L(:,:,3) = R_L3_0; 
% end

rL1_1_1 = R_L1(1,1); rL1_1_2 = R_L1(1,2); rL1_1_3 = R_L1(1,3);
rL1_2_1 = R_L1(2,1); rL1_2_2 = R_L1(2,2); rL1_2_3 = R_L1(2,3);
rL1_3_1 = R_L1(3,1); rL1_3_2 = R_L1(3,2); rL1_3_3 = R_L1(3,3);


rL2_1_1 = R_L2(1,1); rL2_1_2 = R_L2(1,2); rL2_1_3 = R_L2(1,3);
rL2_2_1 = R_L2(2,1); rL2_2_2 = R_L2(2,2); rL2_2_3 = R_L2(2,3);
rL2_3_1 = R_L2(3,1); rL2_3_2 = R_L2(3,2); rL2_3_3 = R_L2(3,3);

rL3_1_1 = R_L3(1,1); rL3_1_2 = R_L3(1,2); rL3_1_3 = R_L3(1,3);
rL3_2_1 = R_L3(2,1); rL3_2_2 = R_L3(2,2); rL3_2_3 = R_L3(2,3);
rL3_3_1 = R_L3(3,1); rL3_3_2 = R_L3(3,2); rL3_3_3 = R_L3(3,3);


newton_iterations = 0;
S=ones(33,1);
while norm(S) > tolerance
    newton_iterations = newton_iterations +1;
    
    %Qd = [M_x;U1_x;U2_x;L1_x;L2_x;P_x;M_y;U1_y;U2_y;L1_y;L2_y;P_y;thetaL1;thetaL2]; 
    M_x = qd(1);
    M_y = qd(2);
    M_z = qd(3);
    U1_x = qd(4);
    U1_y = qd(5);
    U1_z = qd(6);
      L1_x = qd(7);
      L1_y = qd(8);
      L1_z = qd(9);
 thetaL1_x = qd(10);
 thetaL1_y = qd(11);
 thetaL1_z = qd(12);
      U2_x = qd(13);
      U2_y = qd(14);
      U2_z = qd(15);
      L2_x = qd(16);
      L2_y = qd(17);
      L2_z = qd(18);
 thetaL2_x = qd(19);
 thetaL2_y = qd(20);
 thetaL2_z = qd(21);
      U3_x = qd(22);
      U3_y = qd(23);
      U3_z = qd(24);
      L3_x = qd(25);
      L3_y = qd(26);
      L3_z = qd(27);
 thetaL3_x = qd(28);
 thetaL3_y = qd(29);
 thetaL3_z = qd(30);
       P_x = qd(31);
       P_y = qd(32);
       P_z = qd(33);
    
    
    %S = -eval(subs(subs(System,Q,q),t,time));
    S = [...
    ... # Arm 1:  3x3 = 9 constraints
    [M_x;M_y;M_z] + R_A1*[D/2; 0 ;0] - [U1_x; U1_y; U1_z] - R_U1*[0;0;L(1)/2];
    [U1_x; U1_y; U1_z] + R_U1*[0;0;-L(1)/2] - [L1_x; L1_y; L1_z] - R_L1*[0;0;L(2)/2];
    [L1_x; L1_y; L1_z] + R_L1*[0;0;-L(2)/2] - [P_x; P_y; P_z] - R_A1*[L(3)/2;0 ;0];
    ... # Arm 2:  3x3 = 9 constraints
    [M_x;M_y;M_z] + R_A2*[D/2; 0 ;0] - [U2_x; U2_y; U2_z] - R_U2*[0;0;L(1)/2];
    [U2_x; U2_y; U2_z] + R_U2*[0;0;-L(1)/2] - [L2_x; L2_y; L2_z] - R_L2*[0;0;L(2)/2];
    [L2_x; L2_y; L2_z] + R_L2*[0;0;-L(2)/2] - [P_x; P_y; P_z] - R_A2*[L(3)/2;0 ;0];
    ... # Arm 3:  3x3 = 9 constraints
    [M_x;M_y;M_z] + R_A3*[D/2; 0 ;0] - [U3_x; U3_y; U3_z] - R_U3*[0;0;L(1)/2];
    [U3_x; U3_y; U3_z] + R_U3*[0;0;-L(1)/2] - [L3_x; L3_y; L3_z] - R_L3*[0;0;L(2)/2];
    [L3_x; L3_y; L3_z] + R_L3*[0;0;-L(2)/2] - [P_x; P_y; P_z] - R_A3*[L(3)/2;0 ;0];
        ... # Fixed variables:  3 constraints
    [M_x;M_y;M_z];
     ... # Fixed lower link spin in own axis
    [0 1 0]*R_L1.'*R_L1_0*[1;0;0];  % L1_y has no component in L1_x_0
    [0 1 0]*R_L2.'*R_L2_0*[1;0;0]; % L2_y has no component in L2_x_0
    [0 1 0]*R_L3.'*R_L3_0*[1;0;0]; % L3_y has no component in L3_x_0
    ];

    %J =  eval(subs(subs(Jacobian,Q,q),t,time));
    %%function Jacobian_d = Jacobian_dNumeric(L_l,rL1_1_1,rL1_1_2,rL1_2_1,rL1_2_2,rL1_3_1,rL1_3_2,rL2_1_1,rL2_1_2,rL2_2_1,rL2_2_2,rL2_3_1,rL2_3_2,rL3_1_1,rL3_1_2,rL3_2_1,rL3_2_2,rL3_3_1,rL3_3_2)
    %    This function was generated by the Symbolic Math Toolbox version 8.0.
    t2 = L_l.*rL1_1_2.*rL1_2_1.*(1.0./2.0);
    t3 = L_l.*rL1_1_2.*rL1_3_1.*(1.0./2.0);
    t4 = L_l.*rL1_2_2.*rL1_3_1.*(1.0./2.0);
    t5 = L_l.*rL1_1_1.*rL1_2_2.*(1.0./2.0);
    t6 = L_l.*rL1_1_1.*rL1_3_2.*(1.0./2.0);
    t7 = -t2+t5;
    t8 = L_l.*rL1_2_1.*rL1_3_2.*(1.0./2.0);
    t9 = -t3+t6;
    t10 = -t4+t8;
    t11 = L_l.*rL2_1_2.*rL2_2_1.*(1.0./2.0);
    t12 = L_l.*rL2_1_2.*rL2_3_1.*(1.0./2.0);
    t13 = L_l.*rL2_2_2.*rL2_3_1.*(1.0./2.0);
    t14 = L_l.*rL2_1_1.*rL2_2_2.*(1.0./2.0);
    t15 = L_l.*rL2_1_1.*rL2_3_2.*(1.0./2.0);
    t16 = -t11+t14;
    t17 = L_l.*rL2_2_1.*rL2_3_2.*(1.0./2.0);
    t18 = -t12+t15;
    t19 = -t13+t17;
    t20 = L_l.*rL3_1_2.*rL3_2_1.*(1.0./2.0);
    t21 = L_l.*rL3_1_2.*rL3_3_1.*(1.0./2.0);
    t22 = L_l.*rL3_2_2.*rL3_3_1.*(1.0./2.0);
    t23 = L_l.*rL3_1_1.*rL3_2_2.*(1.0./2.0);
    t24 = L_l.*rL3_1_1.*rL3_3_2.*(1.0./2.0);
    t25 = -t20+t23;
    t26 = L_l.*rL3_2_1.*rL3_3_2.*(1.0./2.0);
    t27 = -t21+t24;
    t28 = -t22+t26;
    t29 = sqrt(2.0);
    t30 = sqrt(3.0);
    Jacobian_d = reshape([1.0,0.0,0.0,0.0,0.0,0.0,0.0,0.0,0.0,1.0,0.0,0.0,0.0,0.0,0.0,0.0,0.0,0.0,1.0,0.0,0.0,0.0,0.0,0.0,0.0,0.0,0.0,1.0,0.0,0.0,0.0,0.0,0.0,0.0,1.0,0.0,0.0,0.0,0.0,0.0,0.0,0.0,0.0,1.0,0.0,0.0,0.0,0.0,0.0,0.0,0.0,0.0,1.0,0.0,0.0,0.0,0.0,0.0,0.0,0.0,0.0,1.0,0.0,0.0,0.0,0.0,0.0,0.0,1.0,0.0,0.0,0.0,0.0,0.0,0.0,0.0,0.0,1.0,0.0,0.0,0.0,0.0,0.0,0.0,0.0,0.0,1.0,0.0,0.0,0.0,0.0,0.0,0.0,0.0,0.0,1.0,0.0,0.0,0.0,-1.0,0.0,0.0,1.0,0.0,0.0,0.0,0.0,0.0,0.0,0.0,0.0,0.0,0.0,0.0,0.0,0.0,0.0,0.0,0.0,0.0,0.0,0.0,0.0,0.0,0.0,0.0,0.0,0.0,0.0,0.0,0.0,0.0,0.0,-1.0,0.0,0.0,1.0,0.0,0.0,0.0,0.0,0.0,0.0,0.0,0.0,0.0,0.0,0.0,0.0,0.0,0.0,0.0,0.0,0.0,0.0,0.0,0.0,0.0,0.0,0.0,0.0,0.0,0.0,0.0,0.0,0.0,0.0,-1.0,0.0,0.0,1.0,0.0,0.0,0.0,0.0,0.0,0.0,0.0,0.0,0.0,0.0,0.0,0.0,0.0,0.0,0.0,0.0,0.0,0.0,0.0,0.0,0.0,0.0,0.0,0.0,0.0,0.0,0.0,0.0,0.0,0.0,-1.0,0.0,0.0,1.0,0.0,0.0,0.0,0.0,0.0,0.0,0.0,0.0,0.0,0.0,0.0,0.0,0.0,0.0,0.0,0.0,0.0,0.0,0.0,0.0,0.0,0.0,0.0,0.0,0.0,0.0,0.0,0.0,0.0,0.0,-1.0,0.0,0.0,1.0,0.0,0.0,0.0,0.0,0.0,0.0,0.0,0.0,0.0,0.0,0.0,0.0,0.0,0.0,0.0,0.0,0.0,0.0,0.0,0.0,0.0,0.0,0.0,0.0,0.0,0.0,0.0,0.0,0.0,0.0,-1.0,0.0,0.0,1.0,0.0,0.0,0.0,0.0,0.0,0.0,0.0,0.0,0.0,0.0,0.0,0.0,0.0,0.0,0.0,0.0,0.0,0.0,0.0,0.0,0.0,0.0,0.0,0.0,0.0,0.0,0.0,0.0,t7,t9,0.0,t7,t9,0.0,0.0,0.0,0.0,0.0,0.0,0.0,0.0,0.0,0.0,0.0,0.0,0.0,0.0,0.0,0.0,0.0,0.0,0.0,0.0,0.0,rL1_2_2.*t29.*(-1.0./2.0)+rL1_3_2.*t29.*t30.*(1.0./4.0),0.0,0.0,0.0,0.0,0.0,t2-L_l.*rL1_1_1.*rL1_2_2.*(1.0./2.0),0.0,t10,t2-t5,0.0,t10,0.0,0.0,0.0,0.0,0.0,0.0,0.0,0.0,0.0,0.0,0.0,0.0,0.0,0.0,0.0,0.0,0.0,0.0,0.0,0.0,0.0,rL1_1_2.*t29.*(1.0./2.0)-rL1_3_2.*t29.*(1.0./4.0),0.0,0.0,0.0,0.0,0.0,t3-L_l.*rL1_1_1.*rL1_3_2.*(1.0./2.0),t4-L_l.*rL1_2_1.*rL1_3_2.*(1.0./2.0),0.0,t3-t6,t4-t8,0.0,0.0,0.0,0.0,0.0,0.0,0.0,0.0,0.0,0.0,0.0,0.0,0.0,0.0,0.0,0.0,0.0,0.0,0.0,0.0,0.0,0.0,rL1_2_2.*t29.*(1.0./4.0)-rL1_1_2.*t29.*t30.*(1.0./4.0),0.0,0.0,0.0,0.0,0.0,0.0,0.0,0.0,0.0,0.0,0.0,-1.0,0.0,0.0,1.0,0.0,0.0,0.0,0.0,0.0,0.0,0.0,0.0,0.0,0.0,0.0,0.0,0.0,0.0,0.0,0.0,0.0,0.0,0.0,0.0,0.0,0.0,0.0,0.0,0.0,0.0,0.0,0.0,0.0,0.0,-1.0,0.0,0.0,1.0,0.0,0.0,0.0,0.0,0.0,0.0,0.0,0.0,0.0,0.0,0.0,0.0,0.0,0.0,0.0,0.0,0.0,0.0,0.0,0.0,0.0,0.0,0.0,0.0,0.0,0.0,0.0,0.0,0.0,0.0,-1.0,0.0,0.0,1.0,0.0,0.0,0.0,0.0,0.0,0.0,0.0,0.0,0.0,0.0,0.0,0.0,0.0,0.0,0.0,0.0,0.0,0.0,0.0,0.0,0.0,0.0,0.0,0.0,0.0,0.0,0.0,0.0,0.0,0.0,-1.0,0.0,0.0,1.0,0.0,0.0,0.0,0.0,0.0,0.0,0.0,0.0,0.0,0.0,0.0,0.0,0.0,0.0,0.0,0.0,0.0,0.0,0.0,0.0,0.0,0.0,0.0,0.0,0.0,0.0,0.0,0.0,0.0,0.0,-1.0,0.0,0.0,1.0,0.0,0.0,0.0,0.0,0.0,0.0,0.0,0.0,0.0,0.0,0.0,0.0,0.0,0.0,0.0,0.0,0.0,0.0,0.0,0.0,0.0,0.0,0.0,0.0,0.0,0.0,0.0,0.0,0.0,0.0,-1.0,0.0,0.0,1.0,0.0,0.0,0.0,0.0,0.0,0.0,0.0,0.0,0.0,0.0,0.0,0.0,0.0,0.0,0.0,0.0,0.0,0.0,0.0,0.0,0.0,0.0,0.0,0.0,0.0,0.0,0.0,0.0,t16,t18,0.0,t16,t18,0.0,0.0,0.0,0.0,0.0,0.0,0.0,0.0,0.0,0.0,0.0,0.0,0.0,rL2_2_2.*t29.*(-1.0./2.0)-rL2_3_2.*t29.*t30.*(1.0./4.0),0.0,0.0,0.0,0.0,0.0,0.0,0.0,0.0,0.0,0.0,0.0,0.0,0.0,t11-L_l.*rL2_1_1.*rL2_2_2.*(1.0./2.0),0.0,t19,t11-t14,0.0,t19,0.0,0.0,0.0,0.0,0.0,0.0,0.0,0.0,0.0,0.0,0.0,0.0,0.0,rL2_1_2.*t29.*(1.0./2.0)-rL2_3_2.*t29.*(1.0./4.0),0.0,0.0,0.0,0.0,0.0,0.0,0.0,0.0,0.0,0.0,0.0,0.0,0.0,t12-L_l.*rL2_1_1.*rL2_3_2.*(1.0./2.0),t13-L_l.*rL2_2_1.*rL2_3_2.*(1.0./2.0),0.0,t12-t15,t13-t17,0.0,0.0,0.0,0.0,0.0,0.0,0.0,0.0,0.0,0.0,0.0,0.0,0.0,0.0,rL2_2_2.*t29.*(1.0./4.0)+rL2_1_2.*t29.*t30.*(1.0./4.0),0.0,0.0,0.0,0.0,0.0,0.0,0.0,0.0,0.0,0.0,0.0,0.0,0.0,0.0,0.0,0.0,0.0,0.0,0.0,-1.0,0.0,0.0,1.0,0.0,0.0,0.0,0.0,0.0,0.0,0.0,0.0,0.0,0.0,0.0,0.0,0.0,0.0,0.0,0.0,0.0,0.0,0.0,0.0,0.0,0.0,0.0,0.0,0.0,0.0,0.0,0.0,0.0,0.0,-1.0,0.0,0.0,1.0,0.0,0.0,0.0,0.0,0.0,0.0,0.0,0.0,0.0,0.0,0.0,0.0,0.0,0.0,0.0,0.0,0.0,0.0,0.0,0.0,0.0,0.0,0.0,0.0,0.0,0.0,0.0,0.0,0.0,0.0,-1.0,0.0,0.0,1.0,0.0,0.0,0.0,0.0,0.0,0.0,0.0,0.0,0.0,0.0,0.0,0.0,0.0,0.0,0.0,0.0,0.0,0.0,0.0,0.0,0.0,0.0,0.0,0.0,0.0,0.0,0.0,0.0,0.0,0.0,-1.0,0.0,0.0,1.0,0.0,0.0,0.0,0.0,0.0,0.0,0.0,0.0,0.0,0.0,0.0,0.0,0.0,0.0,0.0,0.0,0.0,0.0,0.0,0.0,0.0,0.0,0.0,0.0,0.0,0.0,0.0,0.0,0.0,0.0,-1.0,0.0,0.0,1.0,0.0,0.0,0.0,0.0,0.0,0.0,0.0,0.0,0.0,0.0,0.0,0.0,0.0,0.0,0.0,0.0,0.0,0.0,0.0,0.0,0.0,0.0,0.0,0.0,0.0,0.0,0.0,0.0,0.0,0.0,-1.0,0.0,0.0,1.0,0.0,0.0,0.0,0.0,0.0,0.0,0.0,0.0,0.0,0.0,0.0,0.0,0.0,0.0,0.0,0.0,0.0,0.0,0.0,0.0,0.0,0.0,0.0,0.0,0.0,0.0,0.0,0.0,t25,t27,0.0,t25,t27,0.0,0.0,0.0,0.0,0.0,rL3_2_2.*t29.*(-1.0./2.0),0.0,0.0,0.0,0.0,0.0,0.0,0.0,0.0,0.0,0.0,0.0,0.0,0.0,0.0,0.0,0.0,0.0,0.0,0.0,0.0,0.0,t20-L_l.*rL3_1_1.*rL3_2_2.*(1.0./2.0),0.0,t28,t20-t23,0.0,t28,0.0,0.0,0.0,0.0,0.0,rL3_1_2.*t29.*(1.0./2.0)+rL3_3_2.*t29.*(1.0./2.0),0.0,0.0,0.0,0.0,0.0,0.0,0.0,0.0,0.0,0.0,0.0,0.0,0.0,0.0,0.0,0.0,0.0,0.0,0.0,0.0,0.0,t21-L_l.*rL3_1_1.*rL3_3_2.*(1.0./2.0),t22-L_l.*rL3_2_1.*rL3_3_2.*(1.0./2.0),0.0,t21-t24,t22-t26,0.0,0.0,0.0,0.0,0.0,0.0,rL3_2_2.*t29.*(-1.0./2.0),0.0,0.0,0.0,0.0,0.0,0.0,-1.0,0.0,0.0,0.0,0.0,0.0,0.0,0.0,0.0,-1.0,0.0,0.0,0.0,0.0,0.0,0.0,0.0,0.0,-1.0,0.0,0.0,0.0,0.0,0.0,0.0,0.0,0.0,0.0,0.0,0.0,0.0,0.0,0.0,0.0,-1.0,0.0,0.0,0.0,0.0,0.0,0.0,0.0,0.0,-1.0,0.0,0.0,0.0,0.0,0.0,0.0,0.0,0.0,-1.0,0.0,0.0,0.0,0.0,0.0,0.0,0.0,0.0,0.0,0.0,0.0,0.0,0.0,0.0,0.0,-1.0,0.0,0.0,0.0,0.0,0.0,0.0,0.0,0.0,-1.0,0.0,0.0,0.0,0.0,0.0,0.0,0.0,0.0,-1.0,0.0,0.0,0.0,0.0,0.0,0.0],[33,33]);

    Delta = Jacobian_d\S;
    qd = Delta+qd;
    % Update the Rotation matrices using a first approximation of the
    % Rodriguez formula
                      % Delta theta_L
    deltaR1=eye(3)+tilde(Delta(10:12));
    deltaR2=eye(3)+tilde(Delta(19:21));
    deltaR3=eye(3)+tilde(Delta(28:30));
    
%     R1=deltaR1*R1;
%     R2=deltaR2*R2;
%     R3=deltaR3*R3;
    R_L1=deltaR1*R_L1;
    rL1_1_1 = R_L1(1,1); rL1_1_2 = R_L1(1,2); rL1_1_3 = R_L1(1,3);
    rL1_2_1 = R_L1(2,1); rL1_2_2 = R_L1(2,2); rL1_2_3 = R_L1(2,3);
    rL1_3_1 = R_L1(3,1); rL1_3_2 = R_L1(3,2); rL1_3_3 = R_L1(3,3);
    
    R_L2=deltaR2*R_L2;
    rL2_1_1 = R_L2(1,1); rL2_1_2 = R_L2(1,2); rL2_1_3 = R_L2(1,3);
    rL2_2_1 = R_L2(2,1); rL2_2_2 = R_L2(2,2); rL2_2_3 = R_L2(2,3);
    rL2_3_1 = R_L2(3,1); rL2_3_2 = R_L2(3,2); rL2_3_3 = R_L2(3,3);
    
    R_L3=deltaR3*R_L3;
    rL3_1_1 = R_L3(1,1); rL3_1_2 = R_L3(1,2); rL3_1_3 = R_L3(1,3);
    rL3_2_1 = R_L3(2,1); rL3_2_2 = R_L3(2,2); rL3_2_3 = R_L3(2,3);
    rL3_3_1 = R_L3(3,1); rL3_3_2 = R_L3(3,2); rL3_3_3 = R_L3(3,3);


    end


end
